simulink subsystem "VehicleAttitude"  (R2024a)
settings: Solver=VariableStepAuto  StartTime=0.0  StopTime=10.0  RelTol=1e-3
libraries: uavmavlinklib x2
settings Model: Creator=gurt1  LastModifiedBy=gurt1

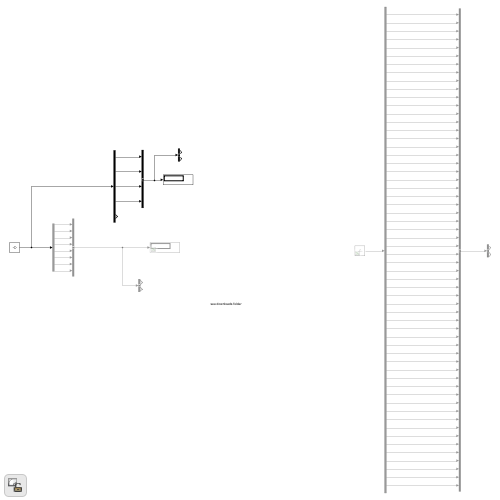
[thumbnail: Simulink's stored preview of the top-level diagram]
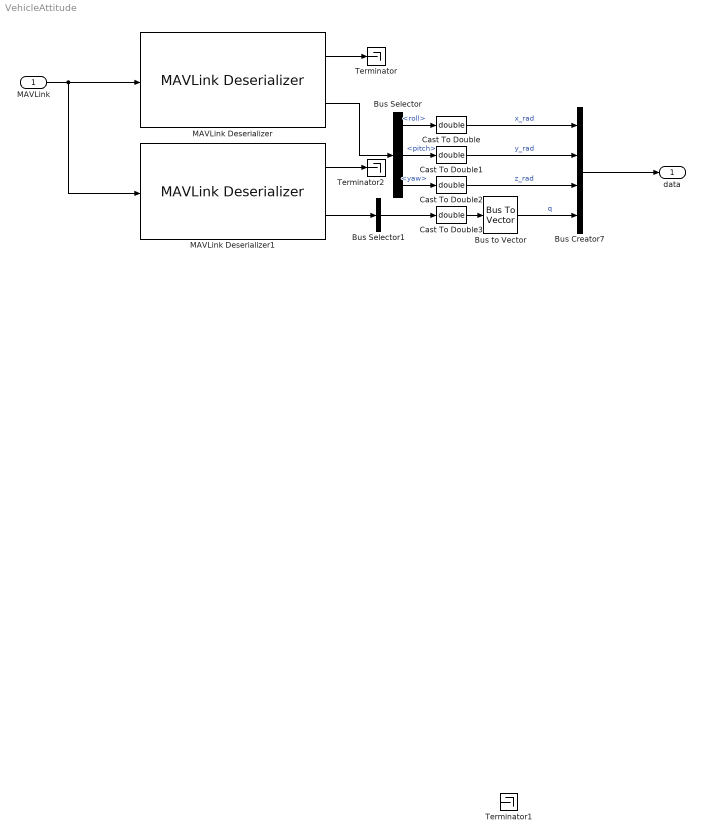
== system VehicleAttitude ==
  MAVLink : Inport
  Bus Creator7 : BusCreator  Inputs=4
  Bus Selector : BusSelector  OutputSignals=Payload.roll,Payload.pitch,Payload.yaw
  Bus Selector1 : BusSelector  OutputSignals=Payload.q1,Payload.q2,Payload.q3,Payload.q4  OutputAsBus=on
  Bus to Vector : BusToVector
  Cast To Double{,1..3} (4 alike) : DataTypeConversion  OutDataTypeStr=double  SaturateOnIntegerOverflow=off  RndMeth=Floor
  MAVLink Deserializer : uavmavlinklib/MAVLink Deserializer  dialectSource=Select from standard MAVLink dialects  dialect=common.xml  dialectCustom=common.xml  version=2  messageType=ATTITUDE  inputDataLength=off  SystemIDFilter=off  systemID=1  ComponentIDFilter=off  componentID=1  queueMsg=off  queueMsgSize=50  dropNum=off
  MAVLink Deserializer1 : uavmavlinklib/MAVLink Deserializer  dialectSource=Select from standard MAVLink dialects  dialect=common.xml  dialectCustom=common.xml  version=2  messageType=ATTITUDE_QUATERNION  inputDataLength=off  SystemIDFilter=off  systemID=1  ComponentIDFilter=off  componentID=1  queueMsg=off  queueMsgSize=50  dropNum=off
  Terminator : Terminator
  Terminator1 : Terminator
  Terminator2 : Terminator
  data : Outport
  wires:
  ? -> ?
  Bus Creator7/1 -> data/1
  MAVLink/1 -> MAVLink Deserializer1/1, MAVLink Deserializer/1
  MAVLink Deserializer/1 -> Terminator/1
  MAVLink Deserializer1/1 -> Terminator2/1
  MAVLink Deserializer/2 -> Bus Selector/1
  MAVLink Deserializer1/2 -> Bus Selector1/1
  Bus Selector1/1 -> Cast To Double3/1
  Bus Selector/1 -> Cast To Double/1  "<roll>"
  Bus Selector/2 -> Cast To Double1/1  "<pitch>"
  Bus Selector/3 -> Cast To Double2/1  "<yaw>"
  Bus to Vector/1 -> Bus Creator7/4  "q"
  Cast To Double3/1 -> Bus to Vector/1
  Cast To Double/1 -> Bus Creator7/1  "x_rad"
  Cast To Double1/1 -> Bus Creator7/2  "y_rad"
  Cast To Double2/1 -> Bus Creator7/3  "z_rad"
